simulink model "zad1"  (R2024a)
settings: Solver=VariableStepAuto  StartTime=0.0  StopTime=25.0  RelTol=1e-3
settings Model: Creator=zv53855  LastModifiedBy=zv53855

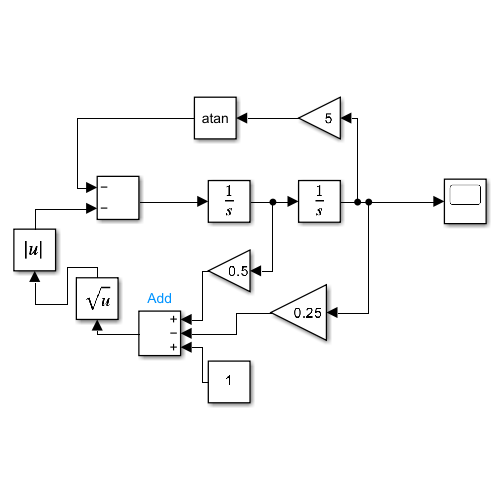
[thumbnail: Simulink's stored preview of the top-level diagram]
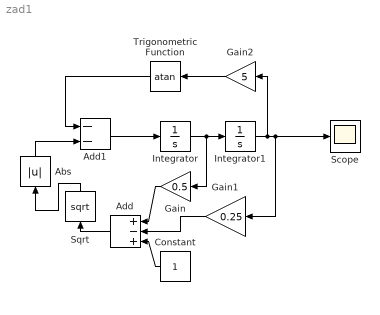
== system zad1 ==
  Abs : Abs  SaturateOnIntegerOverflow=off
  Add : Sum  Inputs=+-+
  Add1 : Sum  Inputs=--
  Constant : Constant
  Gain : Gain  Gain=0.5
  Gain1 : Gain  Gain=0.25
  Gain2 : Gain  Gain=5
  Integrator : Integrator
  Integrator1 : Integrator  InitialCondition=1
  Scope : Scope
  Sqrt : Sqrt
  Trigonometric Function : Trigonometry  Operator=atan
  wires:
  Integrator/1 -> Gain/1, Integrator1/1
  Integrator1/1 -> Gain2/1, Scope/1, Gain1/1
  Gain/1 -> Add/1
  Constant/1 -> Add/3
  Gain1/1 -> Add/2
  Add/1 -> Sqrt/1
  Sqrt/1 -> Abs/1
  Gain2/1 -> Trigonometric Function/1
  Trigonometric Function/1 -> Add1/1
  Add1/1 -> Integrator/1
  Abs/1 -> Add1/2
